simulink model "SingleKernel"  (R2023a)
settings: Solver=VariableStepAuto  StartTime=0.0  StopTime=4096*4  RelTol=1e-3
PreLoadFcn:
  | load taps
undefined symbols (not defined in the file): FIR_SingleStream, S, SingleStream, vsva2197, xcvc1902
libraries: aieBasic x3, dspsrcs4 x2, simulink x1, vmcUtilities x1
settings Model: Creator=abehbood  LastModifiedBy=robg
settings SolverCC: AlgebraicLoopSolver=TrustRegion
settings DebuggingCC: UnconnectedInputMsg=warning  UnconnectedOutputMsg=warning  UnconnectedLineMsg=warning
settings ModelReferenceCC: EnableRefExpFcnMdlSchedulingChecks=on
settings RTWCC: DLArmComputeVersion=19.05

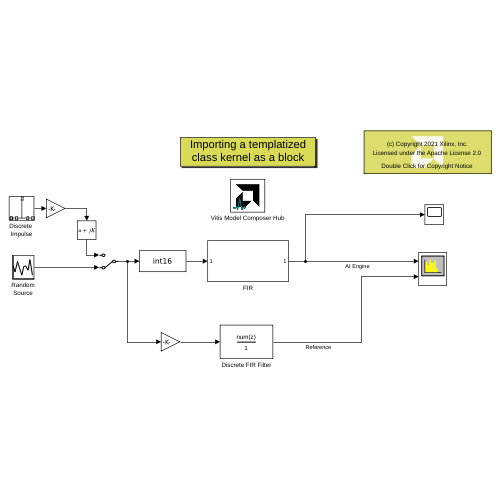
[thumbnail: Simulink's stored preview of the top-level diagram]
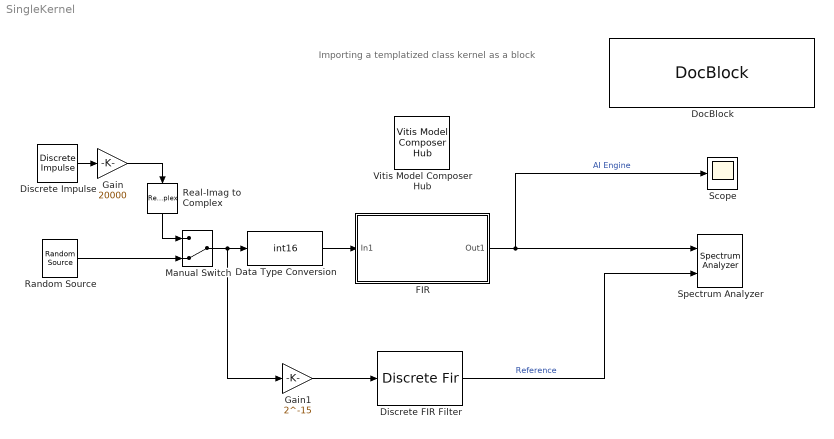
== system SingleKernel ==
  note: Importing a templatized class kernel as a block
  Data Type Conversion : DataTypeConversion  OutDataTypeStr=int16  SaturateOnIntegerOverflow=off  RndMeth=Floor
  Discrete Impulse : dspsrcs4/Discrete  Impulse  Delay=0  SampleTime=1  FrameSample=512  OutputFrames=off  dataType=double  isSigned=on  wordLen=16  udDataType=sfix(16)  fracBitsMode=Best precision  numFracBits=15  OutDataTypeStr=double  LastOutDataTypeStr=double
  Discrete FIR Filter : DiscreteFir  Coefficients=taps'  InputProcessing=Columns as channels (frame based)
  DocBlock : simulink/Model-Wide Utilities/DocBlock  DocumentType=Text  mask(DocBlock){}
      content=|
      | ///////////////////////////////////////////////////////////////////////////
      | // Copyright 2021 Xilinx
      | //
      | // Licensed under the Apache License, Version 2.0 (the "License");
      | // you may not use this file except in compliance with the License.
      | // You may obtain a copy of the License at
      | //
      | // http://www.apache.org/licenses/LICENSE-2.0
      | //
      | // Unless required by applicable law or agreed to in writing, software
      | // distributed under the License is distributed on an "AS IS" BASIS,
      | // WITHOUT WARRANTIES OR CONDITIONS OF ANY KIND, either express or implied.
      | // See the License for the specific language governing permissions and
      | // limitations under the License.
      | ///////////////////////////////////////////////////////////////////////////
      mask Display:
      | xmcDrawBlockIcon();
      | disp(['{\fontsize{10pt}(c) Copyright 2021' ' Xilinx, Inc.}\newline \newline '],'texmode','on');
      | disp('{\fontsize{10pt}Licensed under the Apache License 2.0}','texmode','on');
      | disp('\newline \newline \newline{\fontsize{10pt}Double Click for Copyright Notice}','texmode','on');
  FIR : Subsystem
  Gain : Gain  Gain=20000
  Gain1 : Gain  Gain=2^-15
  Manual Switch : ManualSwitch  CurrentSetting=0
  Random Source : dspsrcs4/Random Source  SrcType=Uniform  NormMethod=Ziggurat  CltLength=12  MinVal=-20000  MaxVal=20000  MeanVal=0  VarVal=1  RepMode=Not repeatable  rawSeed=1  IsInherit=off  SampMode=Discrete  SampTime=1  SampFrame=512  DataType=Double  OutComplex=Complex  OutputFrames=off
  Real-Imag to Complex : RealImagToComplex  Input=Real
  Scope : Scope
  Spectrum Analyzer : SpectrumAnalyzer  NumInputPorts=2  WindowPosition=[24 26 826 443]  Visible=on  Method=Welch  SampleRate=1  Span=1  StartFrequency=-0.5  StopFrequency=0.5  AveragingMethod=Exponential  YLimits=[-9.1704,105.7335]  ShowLegend=on  ChannelNames="[\"\"]"  DefaultConfigurationName=spbscopes.SpectrumAnalyzerBlockCfg
  Vitis Model Composer Hub : vmcUtilities/Vitis Model Composer Hub  Tag=genX  CodeGeneration=off  SubsystemName=FIR  StartColumn=1  NumberOfColumns=1  TargetDirectory=./code  exportDesign=off  analyzeDesign=off  validateDesignOnHw=off  ExportType=HW Code  IpVendor=xilinx.com  IpLibrary=hls  IpVersion=1.0  IpHWLanguage=Verilog  AieCompilerOptions={}  AieSimulatorOptions={}  CreateTestbench=off  TestbenchStackSize=10  RunRtlSim=off  RunCSim=off  RunAieSim=off  AieSimTimeout=50000  RunAieSimProfiling=off  LaunchVitisAnalyzer=off  PlotOutput=off  RunX86Sim=off  X86SimTimeout=10  GenHwImage=off  GenLibadfXo=off  GenHwValidationCode=off  PlatformType=Not Specified  HwSystemType=Baremetal  HwValidationTarget=hw  ProjDevice=xcvc1902-vsva2197-1MP-e-S  ProjDevicePart=xcvc1902-vsva2197-1MP-e-S  AIEType=AIE  SamplePeriod=-1  ClockFrequency=200  DataPathParallelism=1  xilinxfamily=versalaicore  part=xcvc1902  speed=-1MP-e-S  package=vsva2197  directory=./netlist  testbench=off  incr_netlist=off  synthesis_tool=Vivado  clock_wrapper=Clock Enables  dbl_ovrd=According to Block Masks  dcm_input_clock_period=10  sysclk_period=10  simulink_period=1  eval_field=0  LogFileName=''  NThreads=4
  wires:
  Data Type Conversion/1 -> FIR/1(In1)
  FIR/1(Out1) -> Scope/1, Spectrum Analyzer/1  "AI Engine"
  Manual Switch/1 -> Gain1/1, Data Type Conversion/1
  Random Source/1 -> Manual Switch/2
  Discrete Impulse/1 -> Gain/1
  Real-Imag to Complex/1 -> Manual Switch/1
  Gain/1 -> Real-Imag to Complex/1
  Discrete FIR Filter/1 -> Spectrum Analyzer/2  "Reference"
  Gain1/1 -> Discrete FIR Filter/1

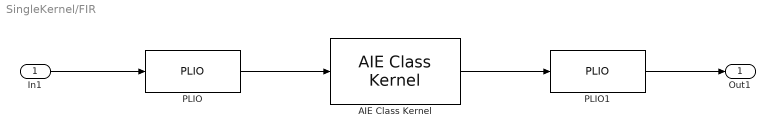
== system SingleKernel/FIR ==
  In1 : Inport
  AIE Class Kernel : aieBasic/AIE Class Kernel  KernelAllAttrs=|  PortNames={'sin'; 'sout'}  PortSerializedTypes={'{P{Tinput_stream{1{t{Scint16}}}}}'; '{P{Toutput_stream{1{t{Scint16}}}}}'}  PortWindowSizes={0.000000000000000000e+00; 0.000000000000000000e+00}  PortWindowMargins={0.000000000000000000e+00; 0.000000000000000000e+00}  PortSynchronicities={'auto', 'auto'}  PortSignalSizes={0.000000000000000000e+00; 5.120000000000000000e+02}  ClassTemplateSpecKind=implicit  ClassTemplateParamNames={'NSamples'; 'ShiftAcc'}  ClassTemplateParamKinds={'nontype'; 'nontype'}  ClassTemplateParamTypes={'int'; 'int'}  ClassTemplateParamValues={'512', '15'}  ClassCtorParamNames={'taps'}  ClassCtorParamSerializedTypes={'{R{Q1{C{Scint16}32}}}'}  ClassCtorParamValues={'[-82-253i;0-204i;11-35i;-198+273i;-642+467i;-1026+333i;-927;-226-73i;643+467i;984+1355i;550+1691i;0+647i;538-1656i;2860-3936i;6313-4587i;9113-2961i;9582;7421+2411i;3936+2860i;1023+1409i;-200-615i;0-1778i;517-1592i;467-643i;-192+140i;-882+287i;-1079;-755-245i;-273-198i;22+30i;63+194i;0+266i]'}  ClassIndex=1  ClassCtorIndex=1  ClassTabVisible=on  ClassTemplateParamsVisible=on  ClassCtorDeclVisible=on  ClassCtorParamsVisible=on  FunctionTabVisible=on  FunctionDecl=|  PortAttrs={ 'input', 'sin', 'input_stream_cint16 *', '', '', '', ''; 'output', 'sout', 'output_stream_cint16 *', '', '', '', '512' }  PortAttrsEnables={'off', 'off', 'off', 'off', 'off', 'off', 'off';'off', 'off', 'off', 'off', 'off', 'off', 'on'}  SampleTime=-1  ClassDeclTypeOptions=|  ClassDecl=|  ClassTemplateParams={ 'NSamples', 'int', '512'; 'ShiftAcc', 'int', '15' }  ClassTemplateParamsEnables={'off', 'off', 'on';'off', 'off', 'on'}  ClassCtorDeclTypeOptions=C[1 1]@t48@FIR_SingleStream(cint16 const ( & taps ) [ 32 ])  ClassCtorDecl=FIR_SingleStream(cint16 const ( & taps ) [ 32 ])  ClassCtorParams={ 'taps', 'cint16 const ( &) [ 32 ]', 'taps' }  KernelHeaderFile=src/aie_kernels/FirSingleStream.h  KernelClassName=SingleStream::FIR_SingleStream  KernelFunction=filter  KernelSourceFile=src/aie_kernels/FirSingleStream.cpp  KernelSearchPaths={}  PreProcOptions={}  blockJsonConstraints=[]
      KernelAllAttrs=|
      | s[12;12;9;9;19;14;21;23;24;21;12;24;26;26;26;27;28;9;21;23;23;23;24;25;14;19;19;29]@FunctionNameDeclFileNamePortNamesPortTypesPortSerializedTypesPortDirectionsPortWindowSizeEnablesPortWindowMarginEnablesPortSynchronicityEnablesPortSignalSizeEnablesFunctionDeclFunctionTemplateSpecKindFunctionTemplateParamNamesFunctionTemplateParamKindsFunctionTemplateParamTypesFunctionTemplateParamValuesFunctionTemplateParamEnablesClassDeclClassTemplateSpecKindClassTemplateParamNamesClassTemplateParamKindsClassTemplateParamTypesClassTemplateParamValuesClassTemplateParamEnablesClassCtorDeclsClassCtorParamNamesClassCtorParamTypesClassCtorParamSerializedTypes[1 1]@C[28 1]@t6@filtert39@../../src/aie_kernels/FirSingleStream.hC[2 1]@t3@sint4@soutC[2 1]@t21@input_stream_cint16 *t22@output_stream_cint16 *C[2 1]@t33@{P{Tinput_stream{1{t{Scint16}}}}}t34@{P{Toutput_stream{1{t{Scint16}}}}}C[2 1]@t5@inputt6@outputC[2 1]@l0@l0@C[2 1]@l0@l0@C[2 1]@l0@l0@C[2 1]@l0@l1@t155@namespace SingleStream {
      | template < int NSamples, int ShiftAcc > 
      | void FIR_SingleStream::
      | filter(input_stream_cint16 * sin, output_stream_cint16 * sout);
      | }t4@nonee[0 1]@e[0 1]@e[0 1]@e[0 1]@e[0 1]@t90@namespace SingleStream {
      | template < int NSamples, int ShiftAcc > class FIR_SingleStream;
      | }t8@implicitC[2 1]@t8@NSamplest8@ShiftAccC[2 1]@t7@nontypet7@nontypeC[2 1]@t3@intt3@intC[2 1]@nnC[2 1]@l1@l1@C[1 1]@t48@FIR_SingleStream(cint16 const ( & taps ) [ 32 ])C[1 1]@C[1 1]@t4@tapsC[1 1]@C[1 1]@t24@cint16 const ( &) [ 32 ]C[1 1]@C[1 1]@t21@{R{Q1{C{Scint16}32}}}
      FunctionDecl=|
      | namespace SingleStream {
      | template < int NSamples, int ShiftAcc > 
      | void FIR_SingleStream::
      | filter(input_stream_cint16 * sin, output_stream_cint16 * sout);
      | }
      ClassDeclTypeOptions=|
      | C[1 1]@t90@namespace SingleStream {
      | template < int NSamples, int ShiftAcc > class FIR_SingleStream;
      | }
      ClassDecl=|
      | namespace SingleStream {
      | template < int NSamples, int ShiftAcc > class FIR_SingleStream;
      | }
  PLIO : aieBasic/PLIO  PlioWidth=64  PlioFreqSpec=off  PlioFreq=250  ColLocation=0  channel=0  blockJsonConstraints=[]  deprecateConstraints=0
  PLIO1 : aieBasic/PLIO  PlioWidth=64  PlioFreqSpec=off  PlioFreq=250  ColLocation=0  channel=0  blockJsonConstraints=[]  deprecateConstraints=0
  Out1 : Outport
  wires:
  In1/1 -> PLIO/1
  PLIO/1 -> AIE Class Kernel/1
  AIE Class Kernel/1 -> PLIO1/1
  PLIO1/1 -> Out1/1
